simulink model "Q12"  (R2017b)
settings: Solver=VariableStepAuto  StartTime=0.0  StopTime=10.0  RelTol=1e-3
settings Model: Creator=HeMaTshop  LastModifiedBy=HeMaTshop

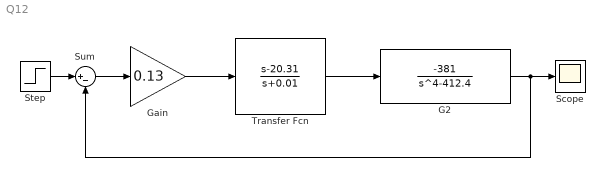
== system Q12 ==
  G2 : TransferFcn  Numerator=[ -381]  Denominator=[1 0 0 0 -412.4]
  Gain : Gain  Gain=0.13
  Scope : Scope
  Step : Step  SampleTime=0
  Sum : Sum  Inputs=|+-
  Transfer Fcn : TransferFcn  Numerator=[1 -20.31]  Denominator=[1 0.01]
  wires:
  Gain/1 -> Transfer Fcn/1
  Transfer Fcn/1 -> G2/1
  Sum/1 -> Gain/1
  Step/1 -> Sum/1
  G2/1 -> Sum/2, Scope/1
